simulink model "ctrl_voltage"  (R2018a)
settings: Solver=FixedStepDiscrete  StartTime=0.0  StopTime=1.6  FixedStep=Ts_Power  RelTol=1e-3  EnableMultiTasking=on
InitFcn:
  | run ctrl_voltage_ini;
values from neighbouring files (symbols this model uses):
  C = 1e-6    (= 1e-06)    [ctrl_voltage_ini.m]    (also in ctrl_voltage_ini_v17b.m)
  L_t = 1.25e-3    (= 0.00125)    [ctrl_voltage_ini.m]    (also in ctrl_voltage_ini_v17b.m)
  params = [R_t;L_t;R_s;L_s;K_p;K_i;C;K_pv;K_iv]    [ctrl_voltage_ini.m]    (also in ctrl_voltage_ini_v17b.m)
  R_d = 20    [ctrl_voltage_ini.m]    (also in ctrl_voltage_ini_v17b.m)
  R_L = 10    [ctrl_voltage_ini.m]    (also in ctrl_voltage_ini_v17b.m)
  R_t = L_t*omega/10    (= 0.0392699081699)    [ctrl_voltage_ini.m]    (also in ctrl_voltage_ini_v17b.m)
  Ts_Control = 50e-6    (= 5e-05)    [ctrl_voltage_ini.m]    (also in ctrl_voltage_ini_v17b.m)
  Ts_Power = 50e-6    (= 5e-05)    [ctrl_voltage_ini.m]    (also in ctrl_voltage_ini_v17b.m)
  v_dc = 730    [ctrl_voltage_ini.m]    (also in ctrl_voltage_ini_v17b.m)
undefined symbols (not defined in the file or in its folder): DiscIntNeverNeededParam
libraries: powerlib x11, powerlib_meascontrol x2
settings Model: Creator=manuelbarragan  LastModifiedBy=manuelbarragan
settings DataIOCC: LimitDataPoints=on  SaveFormat=Array  SignalLoggingSaveFormat=ModelDataLogs
settings OptimizationCC: ExpressionDepthLimit=2147483647  LifeSpan=inf
settings DebuggingCC: UnderspecifiedInitializationDetection=Classic  MergeDetectMultiDrivingBlocksExec=none  SolverPrmCheckMsg=warning  FcnCallInpInsideContextMsg=warning  StateNameClashWarn=warning  SFUnexpectedBacktrackingDiag=warning  SFNoUnconditionalDefaultTransitionDiag=warning  SFExecutionAtInitializationDiag=none
settings HardwareCC: ProdBitPerPointer=32  ProdBitPerSizeT=32  ProdBitPerPtrDiffT=32  ProdLargestAtomicFloat=None  ProdIntDivRoundTo=Undefined  ProdEndianess=Unspecified  ProdWordSize=32  ProdHWDeviceType=32-bit Generic
settings ModelReferenceCC: PropagateSignalLabelsOutOfModel=off
settings CodeAppCC: StateflowObjectComments=on
settings GRTTargetCC: TargetLangStandard=C89/C90 (ANSI)  GeneratePreprocessorConditionals=Disable all  CombineOutputUpdateFcns=off  GRTInterface=on
settings ConfigComp: CovMetricSettings=dw  CovHtmlReporting=on  CovSaveCumulativeToWorkspaceVar=on  CovSaveSingleToWorkspaceVar=on  CovExternalEMLEnable=off
settings SimscapeCC: SimscapeNormalizeSystem=off

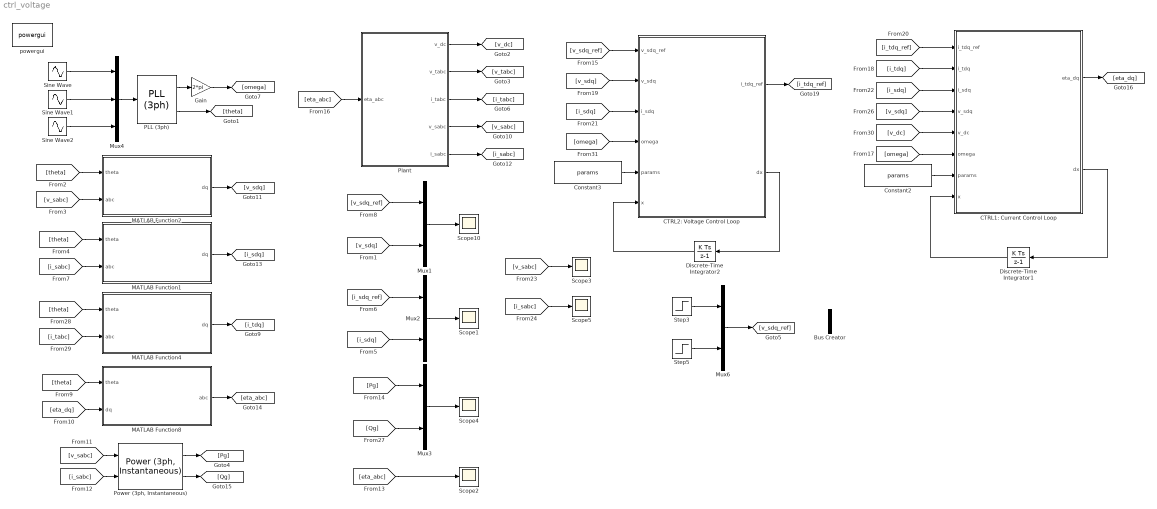
== system ctrl_voltage ==
  Bus Creator : BusCreator  Inputs=2
  CTRL1: Current Control Loop : MATLAB Function  TreatAsAtomicUnit=on
  CTRL2: Voltage Control Loop : MATLAB Function  TreatAsAtomicUnit=on
  Constant2 : Constant  Value=params  SampleTime=Ts_Power
  Constant3 : Constant  Value=params  SampleTime=Ts_Power
  Discrete-Time Integrator1 : DiscreteIntegrator  InitialCondition=[0;0]  SampleTime=Ts_Control  ICPrevOutput=DiscIntNeverNeededParam  ICPrevScaledInput=DiscIntNeverNeededParam
  Discrete-Time Integrator2 : DiscreteIntegrator  InitialCondition=[0;0]  SampleTime=Ts_Control  ICPrevOutput=DiscIntNeverNeededParam  ICPrevScaledInput=DiscIntNeverNeededParam
  Gain : Gain  Gain=2*pi
  MATLAB Function1 : MATLAB Function  TreatAsAtomicUnit=on
  MATLAB Function2 : MATLAB Function  TreatAsAtomicUnit=on
  MATLAB Function4 : MATLAB Function  TreatAsAtomicUnit=on
  MATLAB Function8 : MATLAB Function  TreatAsAtomicUnit=on
  Mux{1..3,6} (4 alike) : Mux  Inputs=2
  Mux4 : Mux  Inputs=3
  PLL (3ph) : powerlib_meascontrol/PLL/PLL (3ph)  Fmin=45  Par_Init=[0, 50]  ParK=[180, 3200, 1]  TcD=1e-4  MaxRateChangeFreq=12  FilterCutOffFreq=25  Ts=Ts_Power  AGC=on
  Plant : Subsystem
  "Power (3ph, Instantaneous)" : powerlib_meascontrol/Measurements/Power (3ph, Instantaneous)
      settings: SourceProductName=Simscape Power Systems
  Scope{1..5,10} (6 alike) : Scope
  Sine Wave : Sin  Amplitude=230*sqrt(2)  Frequency=2*pi*50  SampleTime=0
  Sine Wave1 : Sin  Amplitude=230*sqrt(2)  Frequency=2*pi*50  Phase=-2/3*pi  SampleTime=0
  Sine Wave2 : Sin  Amplitude=230*sqrt(2)  Frequency=2*pi*50  Phase=2/3*pi  SampleTime=0
  Step3 : Step  After=50  SampleTime=0
  Step5 : Step  Time=0.2  After=-230*sqrt(2)  SampleTime=0
  powergui : powerlib/powergui  Priority=1  SimulationMode=Discrete  SampleTime=Ts_Power  frequency=60  Iterations=50  frequencyindice=0  Pbase=100e6  ErrMax=1e-4  UnitsV=kV  UnitsW=MW  buscounter=0  FunctionMessages=off  echomessages=off  EnableUseOfTLC=off  CurrentSourceSwitches=off  DisableSnubberDevices=off  DisableRonSwitches=off  DisableVfSwitches=off  DisplayEquations=off  SolverType=Tustin/Backward Euler (TBE)  Interpol=off  ExternalGateDelay=off  methode=off  Ts=100  x0status=blocks  SPID=off  SwTol=0  HookPort=off  RestoreLinks=warning  ResistiveCurrentMeasurement=off  Frange=[0:2:500]  Ylog=off  Xlog=on  ShowGrid=off  save=off  variable=ZData  structure=0  ZoomFFT=off  StartTime=0.0  cycles=1  DisplayStyle=1  fundamental=60  FreqAxis=off  MaxFrequency=1000  frequencyindicesteady=1  RmsSteady=1  display=off
  wires:
  [theta] -> MATLAB Function2/1(theta)
  [v_sabc] -> MATLAB Function2/2(abc)
  [theta] -> MATLAB Function1/1(theta)
  [i_sabc] -> MATLAB Function1/2(abc)
  MATLAB Function2/1(dq) -> [v_sdq]
  MATLAB Function1/1(dq) -> [i_sdq]
  MATLAB Function8/1(abc) -> [eta_abc]
  [theta] -> MATLAB Function8/1(theta)
  [eta_dq] -> MATLAB Function8/2(dq)
  "Power (3ph, Instantaneous)"/2 -> [Qg]
  [v_sabc] -> "Power (3ph, Instantaneous)"/1
  "Power (3ph, Instantaneous)"/1 -> [Pg]
  [i_sabc] -> "Power (3ph, Instantaneous)"/2
  Mux4/1 -> PLL (3ph)/1
  Mux1/1 -> Scope10/1
  CTRL1: Current Control Loop/2(dx) -> Discrete-Time Integrator1/1
  CTRL1: Current Control Loop/1(eta_dq) -> [eta_dq]
  Mux2/1 -> Scope1/1
  Mux3/1 -> Scope4/1
  [Qg] -> Mux3/2
  [Pg] -> Mux3/1
  Sine Wave/1 -> Mux4/1
  Sine Wave1/1 -> Mux4/2
  Sine Wave2/1 -> Mux4/3
  MATLAB Function4/1(dq) -> [i_tdq]
  [i_tabc] -> MATLAB Function4/2(abc)
  [theta] -> MATLAB Function4/1(theta)
  Constant2/1 -> CTRL1: Current Control Loop/7(params)
  [i_tdq_ref] -> CTRL1: Current Control Loop/1(i_tdq_ref)
  [i_tdq] -> CTRL1: Current Control Loop/2(i_tdq)
  [v_sdq] -> CTRL1: Current Control Loop/4(v_sdq)
  [v_dc] -> CTRL1: Current Control Loop/5(v_dc)
  PLL (3ph)/1 -> Gain/1
  Gain/1 -> [omega]
  PLL (3ph)/2 -> [theta]
  [eta_abc] -> Plant/1(eta_abc)
  Plant/1(v_dc) -> [v_dc]
  Plant/2(v_tabc) -> [v_tabc]
  Plant/3(i_tabc) -> [i_tabc]
  Plant/4(v_sabc) -> [v_sabc]
  Plant/5(i_sabc) -> [i_sabc]
  [omega] -> CTRL1: Current Control Loop/6(omega)
  Discrete-Time Integrator1/1 -> CTRL1: Current Control Loop/8(x)
  [i_sdq] -> Mux2/2
  [i_sdq_ref] -> Mux2/1
  [v_sdq] -> Mux1/2
  [v_sdq_ref] -> Mux1/1
  Step3/1 -> Mux6/1
  Step5/1 -> Mux6/2
  [eta_abc] -> Scope2/1
  [v_sdq_ref] -> CTRL2: Voltage Control Loop/1(v_sdq_ref)
  [v_sdq] -> CTRL2: Voltage Control Loop/2(v_sdq)
  [i_sdq] -> CTRL2: Voltage Control Loop/3(i_sdq)
  [omega] -> CTRL2: Voltage Control Loop/4(omega)
  Constant3/1 -> CTRL2: Voltage Control Loop/5(params)
  CTRL2: Voltage Control Loop/2(dx) -> Discrete-Time Integrator2/1
  Discrete-Time Integrator2/1 -> CTRL2: Voltage Control Loop/6(x)
  CTRL2: Voltage Control Loop/1(i_tdq_ref) -> [i_tdq_ref]
  Mux6/1 -> [v_sdq_ref]
  [i_sdq] -> CTRL1: Current Control Loop/3(i_sdq)
  [v_sabc] -> Scope3/1
  [i_sabc] -> Scope5/1

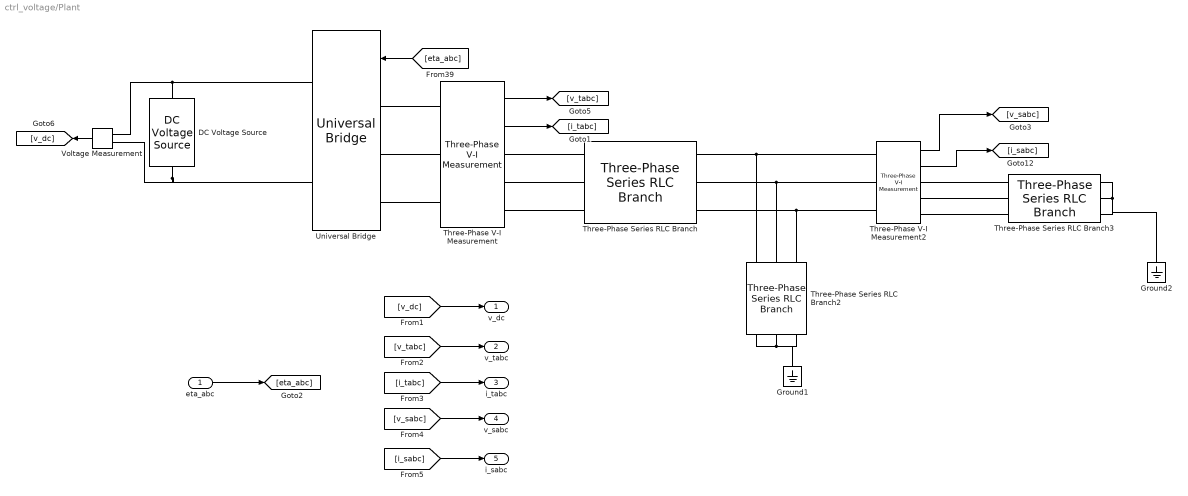
== system ctrl_voltage/Plant ==
  eta_abc : Inport
  DC Voltage Source : powerlib/Electrical Sources/DC Voltage Source  Amplitude=v_dc  Measurements=None
  Ground1 : powerlib/Elements/Ground  LConnTagsString=a
  Ground2 : powerlib/Elements/Ground  LConnTagsString=a
  Three-Phase Series RLC Branch : powerlib/Elements/Three-Phase Series RLC Branch  LConnTagsString=A|B|C  RConnTagsString=A|B|C  BranchType=RL  Resistance=R_t  Inductance=L_t  Capacitance=1e-6  Measurements=None
  Three-Phase Series RLC Branch2 : powerlib/Elements/Three-Phase Series RLC Branch  LConnTagsString=A|B|C  RConnTagsString=A|B|C  BranchType=RC  Resistance=R_d  Inductance=0.1/(100*pi)  Capacitance=C  Measurements=None
  Three-Phase Series RLC Branch3 : powerlib/Elements/Three-Phase Series RLC Branch  LConnTagsString=A|B|C  RConnTagsString=A|B|C  BranchType=R  Resistance=R_L  Inductance=0.1/(100*pi)  Capacitance=1e-6  Measurements=None
  Three-Phase V-I Measurement : powerlib/Measurements/Three-Phase V-I Measurement  VoltageMeasurement=phase-to-ground  SetLabelV=off  LabelV=Vabc  Vpu=off  VpuLL=off  CurrentMeasurement=yes  SetLabelI=off  LabelI=Iabc  Ipu=off  Pbase=100e6  Vbase=500e3  OutputType=Complex  PhasorSimulation=off  PSBequivalent=0
  Three-Phase V-I Measurement2 : powerlib/Measurements/Three-Phase V-I Measurement  VoltageMeasurement=phase-to-ground  SetLabelV=off  LabelV=Vabc  Vpu=off  VpuLL=off  CurrentMeasurement=yes  SetLabelI=off  LabelI=Iabc  Ipu=off  Pbase=100e6  Vbase=500e3  OutputType=Complex  PhasorSimulation=off  PSBequivalent=0
  Universal Bridge : powerlib/Power Electronics/Universal Bridge  Arms=3  SnubberResistance=1e5  SnubberCapacitance=inf  Device=Average-model based VSC  Ron=1e-3  Lon=0  ForwardVoltages="[  0  0  ]"  ForwardVoltage=0  GTOparameters=[ 10e-6 , 20e-6 ]  IGBTparameters=[ 1e-6 , 2e-6 ]  Measurements=None  Measurements_2=None  converterType=Rectifier
  Voltage Measurement : powerlib/Measurements/Voltage Measurement  PhasorSimulation=off  OutputType=Complex  PSBequivalent=0
  v_dc : Outport
  v_tabc : Outport  Port=2
  i_tabc : Outport  Port=3
  v_sabc : Outport  Port=4
  i_sabc : Outport  Port=5
  wires:
  Voltage Measurement/1 -> [v_dc]
  Three-Phase V-I Measurement/2 -> [i_tabc]
  eta_abc/1 -> [eta_abc]
  [eta_abc] -> Universal Bridge/1
  Three-Phase V-I Measurement/1 -> [v_tabc]
  Three-Phase V-I Measurement2/2 -> [i_sabc]
  Three-Phase V-I Measurement2/1 -> [v_sabc]
  [v_dc] -> v_dc/1
  [v_tabc] -> v_tabc/1
  [i_tabc] -> i_tabc/1
  [v_sabc] -> v_sabc/1
  [i_sabc] -> i_sabc/1
  connections:
  Three-Phase Series RLC Branch2/RConn1 -- Three-Phase Series RLC Branch2/RConn3 -- Ground1/LConn1 -- Three-Phase Series RLC Branch2/RConn2
  Three-Phase V-I Measurement/RConn1 -- Three-Phase Series RLC Branch/LConn1
  Three-Phase V-I Measurement/RConn2 -- Three-Phase Series RLC Branch/LConn2
  Three-Phase Series RLC Branch/LConn3 -- Three-Phase V-I Measurement/RConn3
  DC Voltage Source/RConn1 -- Voltage Measurement/LConn1 -- Universal Bridge/RConn1
  Universal Bridge/LConn1 -- Three-Phase V-I Measurement/LConn1
  Universal Bridge/LConn3 -- Three-Phase V-I Measurement/LConn3
  Universal Bridge/LConn2 -- Three-Phase V-I Measurement/LConn2
  Universal Bridge/RConn2 -- Voltage Measurement/LConn2 -- DC Voltage Source/LConn1
  Three-Phase Series RLC Branch3/RConn1 -- Ground2/LConn1 -- Three-Phase Series RLC Branch3/RConn3 -- Three-Phase Series RLC Branch3/RConn2
  Three-Phase V-I Measurement2/LConn1 -- Three-Phase Series RLC Branch2/LConn1 -- Three-Phase Series RLC Branch/RConn1
  Three-Phase V-I Measurement2/LConn2 -- Three-Phase Series RLC Branch2/LConn2 -- Three-Phase Series RLC Branch/RConn2
  Three-Phase V-I Measurement2/LConn3 -- Three-Phase Series RLC Branch2/LConn3 -- Three-Phase Series RLC Branch/RConn3
  Three-Phase V-I Measurement2/RConn1 -- Three-Phase Series RLC Branch3/LConn1
  Three-Phase V-I Measurement2/RConn2 -- Three-Phase Series RLC Branch3/LConn2
  Three-Phase V-I Measurement2/RConn3 -- Three-Phase Series RLC Branch3/LConn3

== matlab function ctrl_voltage/MATLAB Function1 ==
  data: theta input; dq output; abc input
function dq  = fcn(theta,abc)
%#codegen

T_p = 2.0/3.0*[[ cos(theta), cos(theta-2.0/3.0*pi), cos(theta+2.0/3.0*pi)];
               [-sin(theta),-sin(theta-2.0/3.0*pi),-sin(theta+2.0/3.0*pi)]];
           
dq=T_p*abc;

== matlab function ctrl_voltage/CTRL1: Current Control Loop ==
  data: i_tdq_ref input; eta_dq output size=2; i_tdq input; i_sdq input; v_sdq input; v_dc input; dx output; omega input; params input; x input
function [eta_dq,dx] = ctrl_vsc(i_tdq_ref,i_tdq,i_sdq,v_sdq,v_dc,omega,params,x)

% parameters
R_t = params(1);
L_t = params(2);
R_s = params(3);
L_s = params(4);
K_p = params(5);
K_i = params(6);
C = params(7);

%References
i_td_ref = i_tdq_ref(1);
i_tq_ref = i_tdq_ref(2);

%From transformations
%i_td = i_tdq(1); % If current i_tabc is measured
%i_tq = i_tdq(2);
i_sd = i_sdq(1);
i_sq = i_sdq(2);
v_sd = v_sdq(1);
v_sq = v_sdq(2);
i_td = i_sd - C*omega*v_sq; % If current i_tabc is not measured
i_tq = i_sq + C*omega*v_sd;

% from the integrator to the states
xi_itd = x(1);
xi_itq = x(2);


% auxiliar
e_itd = i_td_ref - i_td;
e_itq = i_tq_ref - i_tq;


% derivatives
dxi_itd = e_itd;
dxi_itq = e_itq;


% auxiliar
u_d = K_p*e_itd + K_i*xi_itd;
u_q = K_p*e_itq + K_i*xi_itq;
L = L_t ;
R = R_t ;

% outputs
eta_d = 2/v_dc*(u_d - L*omega*i_tq + v_sd);
eta_q = 2/v_dc*(u_q + L*omega*i_td + v_sq);
eta_dq = [eta_d ; eta_q];


% from derivatives to the integrator
dx = [dxi_itd;dxi_itq];

== matlab function ctrl_voltage/MATLAB Function2 ==
  data: theta input; dq output; abc input
function dq  = fcn(theta,abc)
%#codegen

T_p = 2.0/3.0*[[ cos(theta), cos(theta-2.0/3.0*pi), cos(theta+2.0/3.0*pi)];
               [-sin(theta),-sin(theta-2.0/3.0*pi),-sin(theta+2.0/3.0*pi)]];
           
dq=T_p*abc;

== matlab function ctrl_voltage/CTRL2: Voltage Control Loop ==
  data: v_sdq_ref input; i_tdq_ref output; v_sdq input; i_sdq input; omega input; params input; x input; dx output
function [i_tdq_ref,dx]   = fcn(v_sdq_ref,v_sdq,i_sdq,omega,params,x)

% parameters
C = params(7);
K_pv = params(8);
K_iv = params(9);


%References
v_sd_ref = v_sdq_ref(1);
v_sq_ref = v_sdq_ref(2);

%From transformations
i_sd = i_sdq(1);
i_sq = i_sdq(2);
v_sd = v_sdq(1);
v_sq = v_sdq(2);

% from the integrator to the states
xi_vsd = x(1);
xi_vsq = x(2);

% auxiliar
e_vsd = v_sd_ref - v_sd;
e_vsq = v_sq_ref - v_sq;

% derivatives
dxi_vsd = e_vsd;
dxi_vsq = e_vsq;
dx = [dxi_vsd ; dxi_vsq];

% auxiliar
u_d = K_pv*e_vsd + K_iv*xi_vsd;
u_q = K_pv*e_vsq + K_iv*xi_vsq;

% outputs
i_td_ref=u_d-C*omega*v_sq+i_sd;
i_tq_ref=u_q+C*omega*v_sd+i_sq;

i_tdq_ref = [i_td_ref;i_tq_ref];

== matlab function ctrl_voltage/MATLAB Function4 ==
  data: theta input; dq output; abc input
function dq  = fcn(theta,abc)
%#codegen

T_p = 2.0/3.0*[[ cos(theta), cos(theta-2.0/3.0*pi), cos(theta+2.0/3.0*pi)];
               [-sin(theta),-sin(theta-2.0/3.0*pi),-sin(theta+2.0/3.0*pi)]];
           
dq=T_p*abc;

== matlab function ctrl_voltage/MATLAB Function8 ==
  data: theta input; abc output; dq input
function abc  = fcn(theta,dq)
%#codegen

T_p_inv = [[            cos(theta),            -sin(theta)];
           [ cos(theta-2.0/3.0*pi), -sin(theta-2.0/3.0*pi)];
           [ cos(theta+2.0/3.0*pi), -sin(theta+2.0/3.0*pi)]];
           
abc=T_p_inv*dq;
